simulink model "hw1_SISO_Four_chann_nodamp"  (R2023b)
settings: Solver=ode45  StartTime=0.0  StopTime=10.0  FixedStep=0.001  RelTol=1e-3
values from neighbouring files (symbols this model uses):
  A = 1    [Copy_of_hw1_four_channel_bilateral_teleoperation_params.m]    (also in hw1_four_channel_bilateral_teleoperation_params.m; hw2_2_3_channel_bilateral_teleoperation_params.m; hw3_scattering_teleop_FP_params.m = 1.5; hw3_scattering_teleop_PP_params.m)
  Be = 100    [Copy_of_hw1_four_channel_bilateral_teleoperation_params.m]    (also in hw1_four_channel_bilateral_teleoperation_params.m; hw2_2_3_channel_bilateral_teleoperation_params.m; hw3_scattering_teleop_FP_params.m; hw3_scattering_teleop_PP_params.m)
  Bh = 1    [Copy_of_hw1_four_channel_bilateral_teleoperation_params.m]    (also in hw1_four_channel_bilateral_teleoperation_params.m; hw2_2_3_channel_bilateral_teleoperation_params.m; hw3_scattering_teleop_FP_params.m; hw3_scattering_teleop_PP_params.m)
  Bm = 20*0.8    (= 16)    [Copy_of_hw1_four_channel_bilateral_teleoperation_params.m]    (also in hw1_four_channel_bilateral_teleoperation_params.m; hw2_2_3_channel_bilateral_teleoperation_params.m; hw3_scattering_teleop_FP_params.m; hw3_scattering_teleop_PP_params.m)
  Bs = 4*Bm    (= 64)    [Copy_of_hw1_four_channel_bilateral_teleoperation_params.m]    (also in hw1_four_channel_bilateral_teleoperation_params.m; hw2_2_3_channel_bilateral_teleoperation_params.m; hw3_scattering_teleop_FP_params.m; hw3_scattering_teleop_PP_params.m)
  Dh = 20*0.8    (= 16)    [Copy_of_hw1_four_channel_bilateral_teleoperation_params.m]    (also in hw1_four_channel_bilateral_teleoperation_params.m; hw2_2_3_channel_bilateral_teleoperation_params.m; hw3_scattering_teleop_FP_params.m; hw3_scattering_teleop_PP_params.m)
  Fc = 1    [Copy_of_hw1_four_channel_bilateral_teleoperation_params.m]    (also in hw1_four_channel_bilateral_teleoperation_params.m; hw2_2_3_channel_bilateral_teleoperation_params.m; hw3_scattering_teleop_FP_params.m; hw3_scattering_teleop_PP_params.m)
  Flp = 0.5    [Copy_of_hw1_four_channel_bilateral_teleoperation_params.m]    (also in hw1_four_channel_bilateral_teleoperation_params.m; hw2_2_3_channel_bilateral_teleoperation_params.m; hw3_scattering_teleop_FP_params.m = 0.01; hw3_scattering_teleop_PP_params.m = 0.01)
  Jh = 1    [Copy_of_hw1_four_channel_bilateral_teleoperation_params.m]    (also in hw1_four_channel_bilateral_teleoperation_params.m; hw2_2_3_channel_bilateral_teleoperation_params.m; hw3_scattering_teleop_FP_params.m; hw3_scattering_teleop_PP_params.m)
  Ke = 200    [Copy_of_hw1_four_channel_bilateral_teleoperation_params.m]    (also in hw1_four_channel_bilateral_teleoperation_params.m; hw2_2_3_channel_bilateral_teleoperation_params.m; hw3_scattering_teleop_FP_params.m; hw3_scattering_teleop_PP_params.m)
  Km = 10*1    (= 10)    [Copy_of_hw1_four_channel_bilateral_teleoperation_params.m]    (also in hw1_four_channel_bilateral_teleoperation_params.m; hw2_2_3_channel_bilateral_teleoperation_params.m; hw3_scattering_teleop_FP_params.m; hw3_scattering_teleop_PP_params.m)
  Ks = 4*Km    (= 40)    [Copy_of_hw1_four_channel_bilateral_teleoperation_params.m]    (also in hw1_four_channel_bilateral_teleoperation_params.m; hw2_2_3_channel_bilateral_teleoperation_params.m; hw3_scattering_teleop_FP_params.m; hw3_scattering_teleop_PP_params.m)
  Mm = 0.5    [Copy_of_hw1_four_channel_bilateral_teleoperation_params.m]    (also in hw1_four_channel_bilateral_teleoperation_params.m; hw2_2_3_channel_bilateral_teleoperation_params.m; hw3_scattering_teleop_FP_params.m; hw3_scattering_teleop_PP_params.m)
  Ms = 2    [Copy_of_hw1_four_channel_bilateral_teleoperation_params.m]    (also in hw1_four_channel_bilateral_teleoperation_params.m; hw2_2_3_channel_bilateral_teleoperation_params.m; hw3_scattering_teleop_FP_params.m; hw3_scattering_teleop_PP_params.m)
  Ph = 10*1    (= 10)    [Copy_of_hw1_four_channel_bilateral_teleoperation_params.m]    (also in hw1_four_channel_bilateral_teleoperation_params.m; hw2_2_3_channel_bilateral_teleoperation_params.m; hw3_scattering_teleop_FP_params.m; hw3_scattering_teleop_PP_params.m)
  xe = 5    [Copy_of_hw1_four_channel_bilateral_teleoperation_params.m]    (also in hw1_four_channel_bilateral_teleoperation_params.m = 0.8; hw2_2_3_channel_bilateral_teleoperation_params.m = 2; hw3_scattering_teleop_FP_params.m = 0.8; hw3_scattering_teleop_PP_params.m = 2)
settings Model: Creator=86180  LastModifiedBy=86180

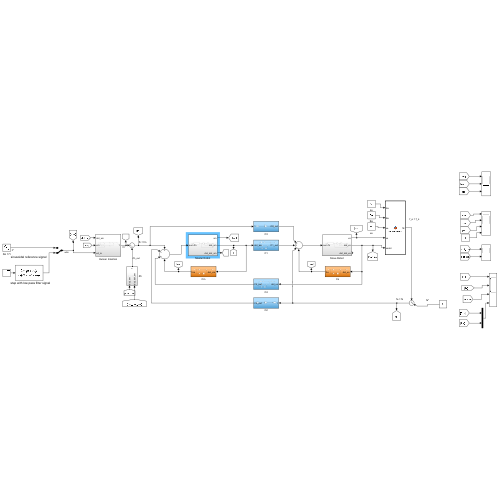
[thumbnail: Simulink's stored preview of the top-level diagram]
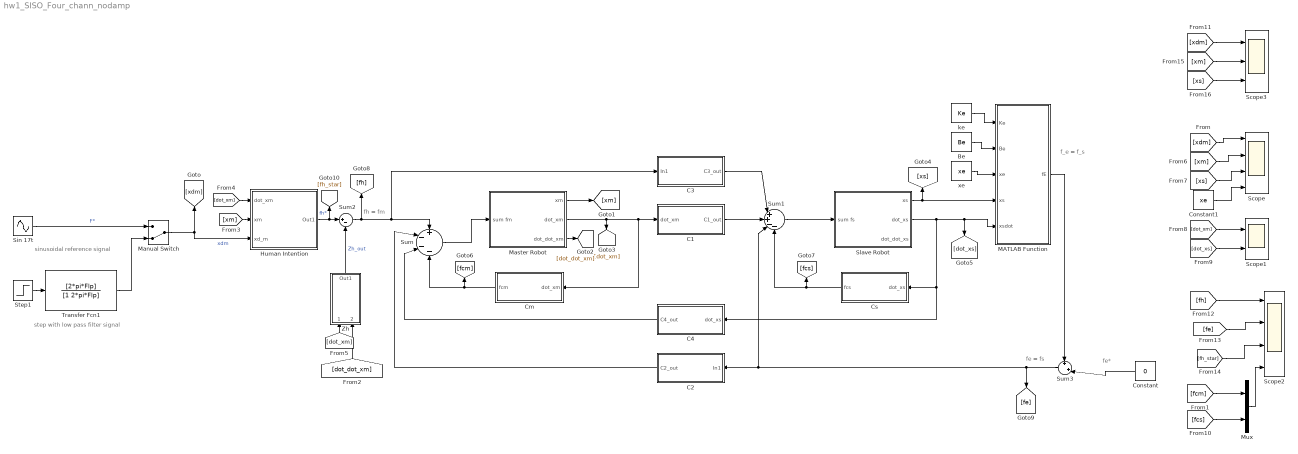
== system hw1_SISO_Four_chann_nodamp ==
  note: f_e = f_s
  note: fe*
  note: fe = fs
  note: fh = fm
  note: sinusoidal reference signal
  note: step with low pass filter signal
  Be : Constant  Value=Be
  C1 : Subsystem
  C2 : Subsystem
  C3 : Subsystem
  C4 : Subsystem
  Cm : Subsystem
  Constant : Constant  Value=0
  Constant1 : Constant  Value=xe
  Cs : Subsystem
  Human Intention : Subsystem
  MATLAB Function : MATLAB Function  TreatAsAtomicUnit=on
  Manual Switch : ManualSwitch  CurrentSetting=0
  Master Robot : Subsystem
  Mux : Mux  Inputs=2
  Scope : Scope  NumInputPorts=4
  Scope1 : Scope  NumInputPorts=2
  Scope2 : Scope  NumInputPorts=4
  Scope3 : Scope  NumInputPorts=3
  Sin 17t : Sin  Amplitude=A  Frequency=2*pi*Fc  SampleTime=0
  Slave Robot : Subsystem
  Step1 : Step  Time=0.5  After=A  SampleTime=0
  Sum : Sum  Inputs=+---
  Sum1 : Sum  Inputs=|++--
  Sum2 : Sum  Inputs=|+-
  Sum3 : Sum  Inputs=+|+|
  Transfer Fcn1 : TransferFcn  Numerator=[2*pi*Flp]  Denominator=[1 2*pi*Flp]
  Zh : Subsystem
  ke : Constant  Value=Ke
  xe : Constant  Value=xe
  wires:
  Manual Switch/1 -> Human Intention/3(xd_m), [xdm]  "xdm"
  Zh/1(Out1) -> Sum2/2  "Zh_out"
  Transfer Fcn1/1 -> Manual Switch/2
  Human Intention/1(Out1) -> [fh_star], Sum2/1  "fh*"
  Sin 17t/1 -> Manual Switch/1  "F*"
  Step1/1 -> Transfer Fcn1/1
  ke/1 -> MATLAB Function/1(Ke)
  xe/1 -> MATLAB Function/3(xe)
  Slave Robot/1(xs) -> MATLAB Function/4(xs), [xs]
  MATLAB Function/1(fE) -> Sum3/1
  Be/1 -> MATLAB Function/2(Be)
  Sum2/1 -> C3/1(In1), Sum/1, [fh]
  Master Robot/2(dot_xm) -> [dot_xm], Cm/1(dot_xm), C1/1(dot_xm)
  Cm/1(fcm) -> [fcm], Sum/4
  C1/1(C1_out) -> Sum1/2
  C4/1(C4_out) -> Sum/3
  C2/1(C2_out) -> Sum/2
  C3/1(C3_out) -> Sum1/1
  Slave Robot/2(dot_xs) -> Cs/1(dot_xs), C4/1(dot_xs), [dot_xs], MATLAB Function/5(xsdot)
  Cs/1(fcs) -> [fcs], Sum1/4
  Sum3/1 -> [fe], Sum1/3, C2/1(In1)
  Constant/1 -> Sum3/2
  [xdm] -> Scope/1
  Master Robot/1(xm) -> [xm]
  Master Robot/3(dot_dot_xm) -> [dot_dot_xm]
  [dot_dot_xm] -> Zh/2(dot_dot_xm)
  [xm] -> Human Intention/2(xm)
  [dot_xm] -> Human Intention/1(dot_xm)
  Sum/1 -> Master Robot/1(sum fm)
  [dot_xm] -> Zh/1(dot_xm)
  [xm] -> Scope/2
  [xs] -> Scope/3
  [dot_xm] -> Scope1/1
  [dot_xs] -> Scope1/2
  Sum1/1 -> Slave Robot/1(sum fs)
  [fh] -> Scope2/1
  [fe] -> Scope2/2
  [fh_star] -> Scope2/3
  [fcs] -> Mux/2
  [fcm] -> Mux/1
  Mux/1 -> Scope2/4
  Constant1/1 -> Scope/4
  [xdm] -> Scope3/1
  [xs] -> Scope3/3
  [xm] -> Scope3/2

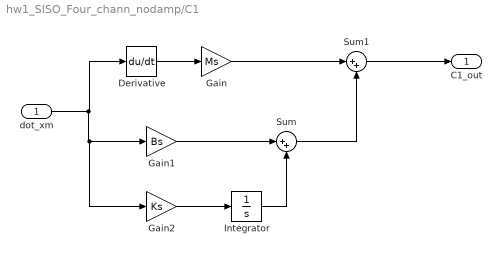
== system hw1_SISO_Four_chann_nodamp/C1 ==
  dot_xm : Inport
  Derivative : Derivative
  Gain : Gain  Gain=Ms
  Gain1 : Gain  Gain=Bs
  Gain2 : Gain  Gain=Ks
  Integrator : Integrator
  Sum : Sum  Inputs=|++
  Sum1 : Sum  Inputs=|++
  C1_out : Outport
  wires:
  dot_xm/1 -> Gain2/1, Gain1/1, Derivative/1
  Derivative/1 -> Gain/1
  Gain2/1 -> Integrator/1
  Gain1/1 -> Sum/1
  Integrator/1 -> Sum/2
  Sum/1 -> Sum1/2
  Gain/1 -> Sum1/1
  Sum1/1 -> C1_out/1

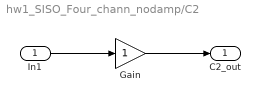
== system hw1_SISO_Four_chann_nodamp/C2 ==
  In1 : Inport
  Gain : Gain
  C2_out : Outport
  wires:
  In1/1 -> Gain/1
  Gain/1 -> C2_out/1

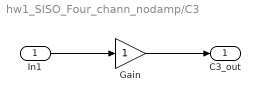
== system hw1_SISO_Four_chann_nodamp/C3 ==
  In1 : Inport
  Gain : Gain
  C3_out : Outport
  wires:
  In1/1 -> Gain/1
  Gain/1 -> C3_out/1

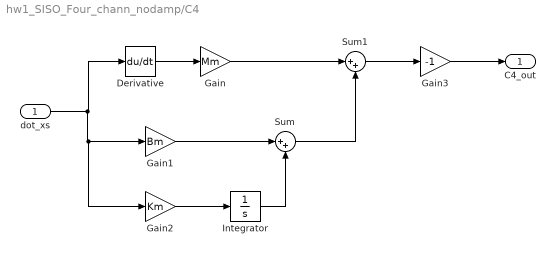
== system hw1_SISO_Four_chann_nodamp/C4 ==
  dot_xs : Inport
  Derivative : Derivative
  Gain : Gain  Gain=Mm
  Gain1 : Gain  Gain=Bm
  Gain2 : Gain  Gain=Km
  Gain3 : Gain  Gain=-1
  Integrator : Integrator
  Sum : Sum  Inputs=|++
  Sum1 : Sum  Inputs=|++
  C4_out : Outport
  wires:
  dot_xs/1 -> Gain2/1, Gain1/1, Derivative/1
  Derivative/1 -> Gain/1
  Gain2/1 -> Integrator/1
  Gain1/1 -> Sum/1
  Integrator/1 -> Sum/2
  Sum/1 -> Sum1/2
  Gain/1 -> Sum1/1
  Sum1/1 -> Gain3/1
  Gain3/1 -> C4_out/1

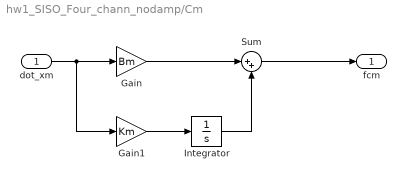
== system hw1_SISO_Four_chann_nodamp/Cm ==
  dot_xm : Inport
  Gain : Gain  Gain=Bm
  Gain1 : Gain  Gain=Km
  Integrator : Integrator
  Sum : Sum  Inputs=|++
  fcm : Outport
  wires:
  dot_xm/1 -> Gain1/1, Gain/1
  Gain1/1 -> Integrator/1
  Gain/1 -> Sum/1
  Integrator/1 -> Sum/2
  Sum/1 -> fcm/1

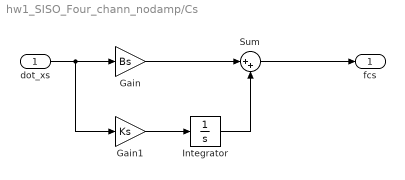
== system hw1_SISO_Four_chann_nodamp/Cs ==
  dot_xs : Inport
  Gain : Gain  Gain=Bs
  Gain1 : Gain  Gain=Ks
  Integrator : Integrator
  Sum : Sum  Inputs=|++
  fcs : Outport
  wires:
  dot_xs/1 -> Gain1/1, Gain/1
  Gain1/1 -> Integrator/1
  Gain/1 -> Sum/1
  Integrator/1 -> Sum/2
  Sum/1 -> fcs/1

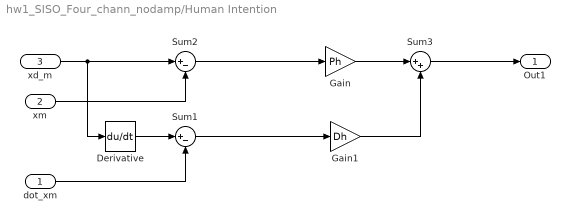
== system hw1_SISO_Four_chann_nodamp/Human Intention ==
  dot_xm : Inport
  xm : Inport  Port=2
  xd_m : Inport  Port=3
  Derivative : Derivative
  Gain : Gain  Gain=Ph
  Gain1 : Gain  Gain=Dh
  Sum1 : Sum  Inputs=|+-
  Sum2 : Sum  Inputs=|+-
  Sum3 : Sum  Inputs=|++
  Out1 : Outport
  wires:
  xm/1 -> Sum2/2
  dot_xm/1 -> Sum1/2
  Sum2/1 -> Gain/1
  Sum1/1 -> Gain1/1
  Gain1/1 -> Sum3/2
  Gain/1 -> Sum3/1
  Sum3/1 -> Out1/1
  xd_m/1 -> Derivative/1, Sum2/1
  Derivative/1 -> Sum1/1

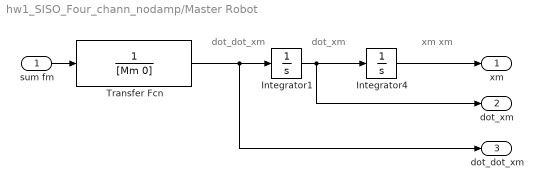
== system hw1_SISO_Four_chann_nodamp/Master Robot ==
  note: dot_dot_xm
  note: dot_xm
  note: xm
      | xm
  sum fm : Inport
  Integrator1 : Integrator
  Integrator4 : Integrator
  Transfer Fcn : TransferFcn  Denominator=[Mm 0]
  xm : Outport
  dot_xm : Outport  Port=2
  dot_dot_xm : Outport  Port=3
  wires:
  Integrator4/1 -> xm/1
  Integrator1/1 -> dot_xm/1, Integrator4/1
  Transfer Fcn/1 -> dot_dot_xm/1, Integrator1/1
  sum fm/1 -> Transfer Fcn/1

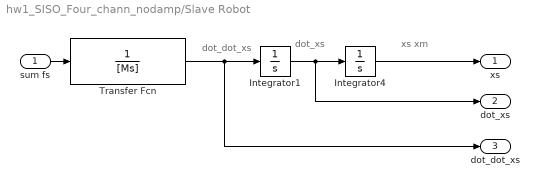
== system hw1_SISO_Four_chann_nodamp/Slave Robot ==
  note: dot_dot_xs
  note: dot_xs
  note: xs
      | xm
  sum fs : Inport
  Integrator1 : Integrator
  Integrator4 : Integrator
  Transfer Fcn : TransferFcn  Denominator=[Ms]
  xs : Outport
  dot_xs : Outport  Port=2
  dot_dot_xs : Outport  Port=3
  wires:
  Integrator4/1 -> xs/1
  Integrator1/1 -> dot_xs/1, Integrator4/1
  Transfer Fcn/1 -> dot_dot_xs/1, Integrator1/1
  sum fs/1 -> Transfer Fcn/1

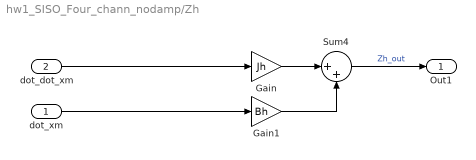
== system hw1_SISO_Four_chann_nodamp/Zh ==
  dot_xm : Inport
  dot_dot_xm : Inport  Port=2
  Gain : Gain  Gain=Jh
  Gain1 : Gain  Gain=Bh
  Sum4 : Sum  Inputs=|++
  Out1 : Outport
  wires:
  dot_dot_xm/1 -> Gain/1
  Gain1/1 -> Sum4/2
  Gain/1 -> Sum4/1
  Sum4/1 -> Out1/1  "Zh_out"
  dot_xm/1 -> Gain1/1

== matlab function hw1_SISO_Four_chann_nodamp/MATLAB Function ==
  data: Ke input; fE output; Be input; xe input; xs input; xsdot input
function fE = environment(Ke, Be, xe, xs, xsdot)
    if xs > xe
        fE = Ke * (xs - xe) + Be * xsdot; % Plot both contributions Ke and Be
    else
        fE = 0;
    end
end
